simulink model "TETAsf"  (R2017b)
settings: Solver=VariableStepAuto  StartTime=0.0  StopTime=60  RelTol=1e-3
libraries: simulink_extras x4
settings Model: Creator=Iman  LastModifiedBy=Iman

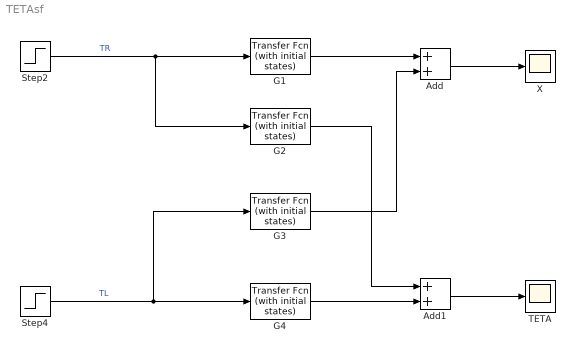
== system TETAsf ==
  Add : Sum
  Add1 : Sum
  G1 : simulink_extras/Additional Linear/Transfer Fcn (with initial states)  N=[104.5 -2150 -3.368e04 -6.03e04]  D=[1 2564 3.781e04 1.506e05 7.832e04 0]  X0=0
  G2 : simulink_extras/Additional Linear/Transfer Fcn (with initial states)  N=[-1374 -8.86e04 -6.695e05]  D=[1 2564 3.781e04 1.506e05 7.832e04]  X0=0
  G3 : simulink_extras/Additional Linear/Transfer Fcn (with initial states)  N=[104.5 -2506 -2.32e04 -3.682e04]  D=[1 2564 3.781e04 1.506e05 7.832e04 0]  X0=0
  G4 : simulink_extras/Additional Linear/Transfer Fcn (with initial states)  N=[-1374 -8.393e04 -4.088e05]  D=[1 2564 3.781e04 1.506e05 7.832e04]  X0=0
  Step2 : Step  Time=0  SampleTime=0.1
  Step4 : Step  Time=0  SampleTime=0.1
  TETA : Scope
  X : Scope
  wires:
  Step4/1 -> G3/1, G4/1  "TL"
  Step2/1 -> G2/1, G1/1  "TR"
  G4/1 -> Add1/2
  G3/1 -> Add/2
  G2/1 -> Add1/1
  Add1/1 -> TETA/1
  Add/1 -> X/1
  G1/1 -> Add/1
